simulink model "ccc_core"  (Simulink 7.4)
settings: Solver=ode45  StartTime=0.0  StopTime=10000  RelTol=1e-3
libraries: xbsIndex_r4 x236, cfa_library x64, casper_library_misc x7
(part 3 of 5)

== system ccc_core/ccc_core/real_bram_vacc ==
  new_acc : Inport  OutDataType=sfix(16)  OutScaling=2^0
  din : Inport  Port=2  OutDataType=sfix(16)  OutScaling=2^0
  Adder : xbsIndex_r4/AddSub  mode=Addition  use_carryin=off  use_carryout=off  en=off  latency=add_latency  precision=User Defined  arith_type="Signed  (2's comp)"  n_bits=n_bits  bin_pt=bin_pt  quantization=Truncate  overflow=Wrap  dbl_ovrd=off  use_behavioral_HDL=off  hw_selection=Fabric  pipelined=on  use_rpm=on  block_type=addsub
      settings: xl_area=[0, 0, 0, 0, 0, 0, 0]  block_version=10.1.3
  Constant : xbsIndex_r4/Constant  arith_type=Signed (2's comp)  const=0  n_bits=n_bits  bin_pt=bin_pt  explicit_period=on  period=1  equ=P=C  opselect=C  inp2=PCIN>>17  opr=+  inp1=P  carry=CIN  dbl_ovrd=off  block_type=constant
  Mux : xbsIndex_r4/Mux  inputs=2  en=off  latency=0  precision=Full  arith_type="Signed  (2's comp)"  n_bits=8  bin_pt=2  quantization=Truncate  overflow=Wrap  dbl_ovrd=off  block_type=mux
      settings: xl_area=[0, 0, 0, 0, 0, 0, 0]
  delay_bram : Subsystem  mask(delay_bram){DelayLen=vec_len - add_latency, bram_latency=add_latency}
      mask prompts: DelayLen "Delay By:"; bram_latency "BRAM Latency"
      mask help: A delay block that uses BRAM for its storage.
      mask init:
      | if (DelayLen <= bram_latency)
      | 	error('delay value must be greater than BRAM Latency');
      | end
      | BitWidth = max(ceil(log2(DelayLen)), 2);
      mask Help: eval('xlWeb(''http://casper.berkeley.edu/wiki/Delay_bram'')')
  pulse_ext : Subsystem  mask(pulse_ext){pulse_len=vec_len}
      mask prompts: pulse_len "Length of Pulse"
      mask help:
      | Extends a boolean signal to be high for the specified number of clocks after
      | the last high input.
      mask init:
      | bits = ceil(log2(pulse_len+1));
      mask Help: eval('xlWeb(''http://casper.berkeley.edu/wiki/Pulse_ext'')')
  dout : Outport  OutDataType=sfix(16)  OutScaling=2^0
  valid : Outport  Port=2  OutDataType=sfix(16)  OutScaling=2^0
  wires:
  Adder/1 -> delay_bram/1(In1)
  delay_bram/1(Out1) -> dout/1, Mux/2
  new_acc/1 -> pulse_ext/1(in)
  din/1 -> Adder/1
  pulse_ext/1(out) -> Mux/1, valid/1
  Mux/1 -> Adder/2
  Constant/1 -> Mux/3

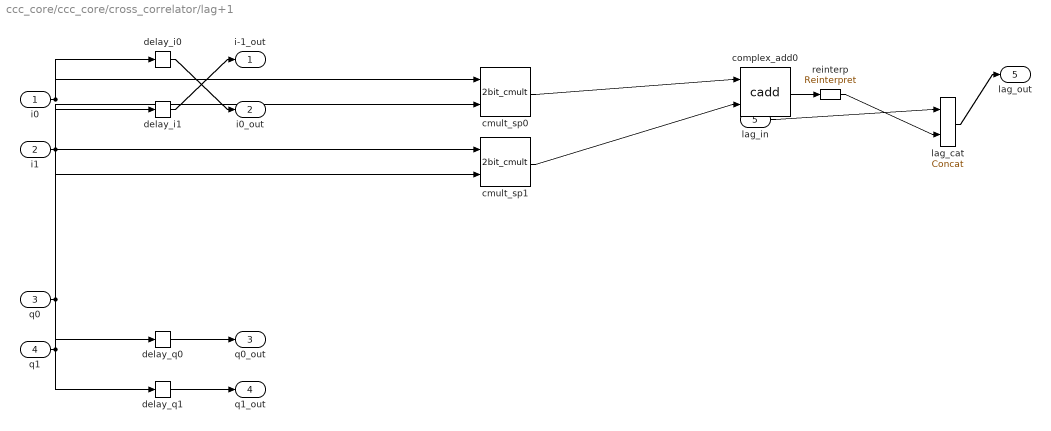
== system ccc_core/ccc_core/cross_correlator/lag+1 ==
  i0 : Inport
  i1 : Inport  Port=2
  q0 : Inport  Port=3
  q1 : Inport  Port=4
  lag_in : Inport  Port=5
  cmult_sp0 : cfa_library/2bit_cmult  SystemSampleTime=-1  add_delay=2
  cmult_sp1 : cfa_library/2bit_cmult  SystemSampleTime=-1  add_delay=2
  complex_add0 : cfa_library/cadd  SystemSampleTime=-1  input_bit_width=6  input_bin_pt=0  add_delay=2
  delay_i0 : xbsIndex_r4/Delay  en=off  latency=2  dbl_ovrd=off  reg_retiming=off  block_type=delay
      settings: block_version=11.4
  delay_i1 : xbsIndex_r4/Delay  en=off  latency=3  dbl_ovrd=off  reg_retiming=off  block_type=delay
      settings: block_version=11.4
  delay_q0 : xbsIndex_r4/Delay  en=off  latency=2  dbl_ovrd=off  reg_retiming=off  block_type=delay
      settings: block_version=11.4
  delay_q1 : xbsIndex_r4/Delay  en=off  latency=2  dbl_ovrd=off  reg_retiming=off  block_type=delay
      settings: block_version=11.4
  lag_cat : xbsIndex_r4/Concat  num_inputs=2  dbl_ovrd=off  block_type=concat
  reinterp : xbsIndex_r4/Reinterpret  force_arith_type=on  arith_type=Unsigned  force_bin_pt=on  bin_pt=0  block_type=reinterpret
      settings: infoedit="Changes signal type without altering the binary representation.   You can changed the signal between signed and unsigned, and relocate the binary point.<br><br>Hardware notes: In hardware this block costs nothing.<br><br>Example:  Suppose the input is 6 bits wide, signed, with 2 fractional bits, and the output is forced to unsigned with 0 fractional bits.  Then an input of -2.0 (1110.00 in binary 2's complement) becomes an output of 56 (111000 in binary)."
  i-1_out : Outport
  i0_out : Outport  Port=2
  q0_out : Outport  Port=3
  q1_out : Outport  Port=4
  lag_out : Outport  Port=5
  wires:
  i0/1 -> cmult_sp0/1, delay_i0/1
  q0/1 -> cmult_sp0/2, delay_q0/1
  i1/1 -> cmult_sp1/1, delay_i1/1
  q1/1 -> cmult_sp1/2, delay_q1/1
  cmult_sp0/1 -> complex_add0/1
  cmult_sp1/1 -> complex_add0/2
  delay_i0/1 -> i0_out/1
  delay_q0/1 -> q0_out/1
  delay_i1/1 -> i-1_out/1
  delay_q1/1 -> q1_out/1
  lag_in/1 -> lag_cat/1
  complex_add0/1 -> reinterp/1
  reinterp/1 -> lag_cat/2
  lag_cat/1 -> lag_out/1

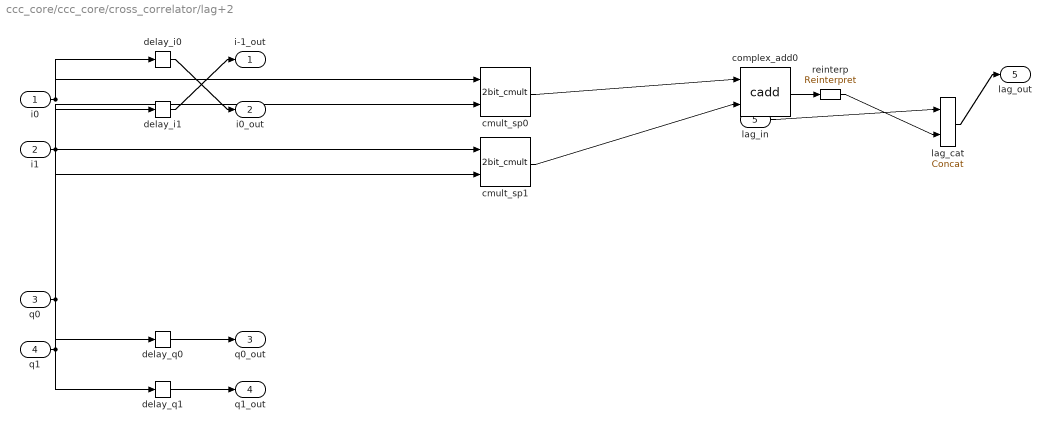
== system ccc_core/ccc_core/cross_correlator/lag+2 ==
  i0 : Inport
  i1 : Inport  Port=2
  q0 : Inport  Port=3
  q1 : Inport  Port=4
  lag_in : Inport  Port=5
  cmult_sp0 : cfa_library/2bit_cmult  SystemSampleTime=-1  add_delay=2
  cmult_sp1 : cfa_library/2bit_cmult  SystemSampleTime=-1  add_delay=2
  complex_add0 : cfa_library/cadd  SystemSampleTime=-1  input_bit_width=6  input_bin_pt=0  add_delay=2
  delay_i0 : xbsIndex_r4/Delay  en=off  latency=2  dbl_ovrd=off  reg_retiming=off  block_type=delay
      settings: block_version=11.4
  delay_i1 : xbsIndex_r4/Delay  en=off  latency=3  dbl_ovrd=off  reg_retiming=off  block_type=delay
      settings: block_version=11.4
  delay_q0 : xbsIndex_r4/Delay  en=off  latency=2  dbl_ovrd=off  reg_retiming=off  block_type=delay
      settings: block_version=11.4
  delay_q1 : xbsIndex_r4/Delay  en=off  latency=2  dbl_ovrd=off  reg_retiming=off  block_type=delay
      settings: block_version=11.4
  lag_cat : xbsIndex_r4/Concat  num_inputs=2  dbl_ovrd=off  block_type=concat
  reinterp : xbsIndex_r4/Reinterpret  force_arith_type=on  arith_type=Unsigned  force_bin_pt=on  bin_pt=0  block_type=reinterpret
      settings: infoedit="Changes signal type without altering the binary representation.   You can changed the signal between signed and unsigned, and relocate the binary point.<br><br>Hardware notes: In hardware this block costs nothing.<br><br>Example:  Suppose the input is 6 bits wide, signed, with 2 fractional bits, and the output is forced to unsigned with 0 fractional bits.  Then an input of -2.0 (1110.00 in binary 2's complement) becomes an output of 56 (111000 in binary)."
  i-1_out : Outport
  i0_out : Outport  Port=2
  q0_out : Outport  Port=3
  q1_out : Outport  Port=4
  lag_out : Outport  Port=5
  wires:
  i0/1 -> cmult_sp0/1, delay_i0/1
  q0/1 -> cmult_sp0/2, delay_q0/1
  i1/1 -> cmult_sp1/1, delay_i1/1
  q1/1 -> cmult_sp1/2, delay_q1/1
  cmult_sp0/1 -> complex_add0/1
  cmult_sp1/1 -> complex_add0/2
  delay_i0/1 -> i0_out/1
  delay_q0/1 -> q0_out/1
  delay_i1/1 -> i-1_out/1
  delay_q1/1 -> q1_out/1
  lag_in/1 -> lag_cat/1
  complex_add0/1 -> reinterp/1
  reinterp/1 -> lag_cat/2
  lag_cat/1 -> lag_out/1

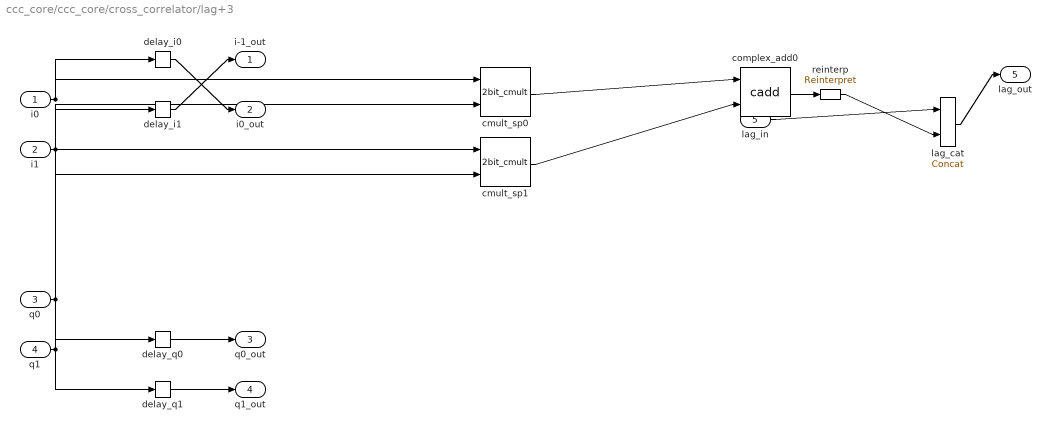
== system ccc_core/ccc_core/cross_correlator/lag+3 ==
  i0 : Inport
  i1 : Inport  Port=2
  q0 : Inport  Port=3
  q1 : Inport  Port=4
  lag_in : Inport  Port=5
  cmult_sp0 : cfa_library/2bit_cmult  SystemSampleTime=-1  add_delay=2
  cmult_sp1 : cfa_library/2bit_cmult  SystemSampleTime=-1  add_delay=2
  complex_add0 : cfa_library/cadd  SystemSampleTime=-1  input_bit_width=6  input_bin_pt=0  add_delay=2
  delay_i0 : xbsIndex_r4/Delay  en=off  latency=2  dbl_ovrd=off  reg_retiming=off  block_type=delay
      settings: block_version=11.4
  delay_i1 : xbsIndex_r4/Delay  en=off  latency=3  dbl_ovrd=off  reg_retiming=off  block_type=delay
      settings: block_version=11.4
  delay_q0 : xbsIndex_r4/Delay  en=off  latency=2  dbl_ovrd=off  reg_retiming=off  block_type=delay
      settings: block_version=11.4
  delay_q1 : xbsIndex_r4/Delay  en=off  latency=2  dbl_ovrd=off  reg_retiming=off  block_type=delay
      settings: block_version=11.4
  lag_cat : xbsIndex_r4/Concat  num_inputs=2  dbl_ovrd=off  block_type=concat
  reinterp : xbsIndex_r4/Reinterpret  force_arith_type=on  arith_type=Unsigned  force_bin_pt=on  bin_pt=0  block_type=reinterpret
      settings: infoedit="Changes signal type without altering the binary representation.   You can changed the signal between signed and unsigned, and relocate the binary point.<br><br>Hardware notes: In hardware this block costs nothing.<br><br>Example:  Suppose the input is 6 bits wide, signed, with 2 fractional bits, and the output is forced to unsigned with 0 fractional bits.  Then an input of -2.0 (1110.00 in binary 2's complement) becomes an output of 56 (111000 in binary)."
  i-1_out : Outport
  i0_out : Outport  Port=2
  q0_out : Outport  Port=3
  q1_out : Outport  Port=4
  lag_out : Outport  Port=5
  wires:
  i0/1 -> cmult_sp0/1, delay_i0/1
  q0/1 -> cmult_sp0/2, delay_q0/1
  i1/1 -> cmult_sp1/1, delay_i1/1
  q1/1 -> cmult_sp1/2, delay_q1/1
  cmult_sp0/1 -> complex_add0/1
  cmult_sp1/1 -> complex_add0/2
  delay_i0/1 -> i0_out/1
  delay_q0/1 -> q0_out/1
  delay_i1/1 -> i-1_out/1
  delay_q1/1 -> q1_out/1
  lag_in/1 -> lag_cat/1
  complex_add0/1 -> reinterp/1
  reinterp/1 -> lag_cat/2
  lag_cat/1 -> lag_out/1

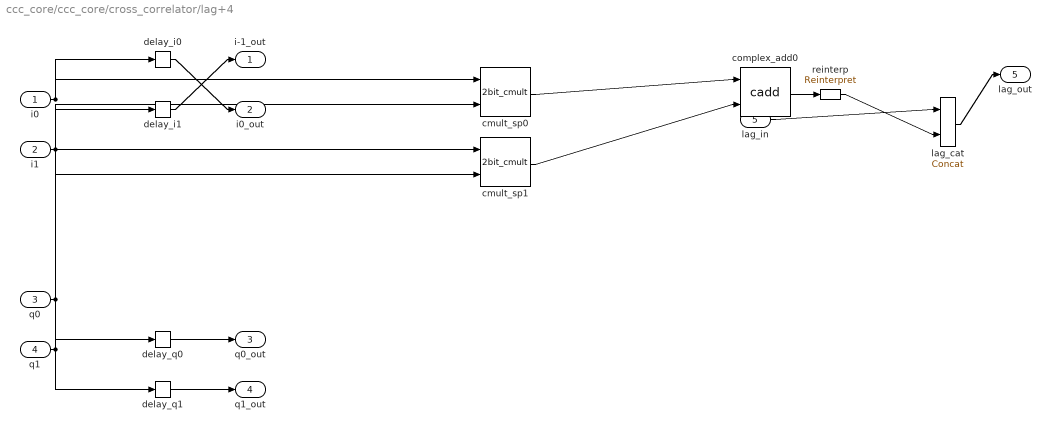
== system ccc_core/ccc_core/cross_correlator/lag+4 ==
  i0 : Inport
  i1 : Inport  Port=2
  q0 : Inport  Port=3
  q1 : Inport  Port=4
  lag_in : Inport  Port=5
  cmult_sp0 : cfa_library/2bit_cmult  SystemSampleTime=-1  add_delay=2
  cmult_sp1 : cfa_library/2bit_cmult  SystemSampleTime=-1  add_delay=2
  complex_add0 : cfa_library/cadd  SystemSampleTime=-1  input_bit_width=6  input_bin_pt=0  add_delay=2
  delay_i0 : xbsIndex_r4/Delay  en=off  latency=2  dbl_ovrd=off  reg_retiming=off  block_type=delay
      settings: block_version=11.4
  delay_i1 : xbsIndex_r4/Delay  en=off  latency=3  dbl_ovrd=off  reg_retiming=off  block_type=delay
      settings: block_version=11.4
  delay_q0 : xbsIndex_r4/Delay  en=off  latency=2  dbl_ovrd=off  reg_retiming=off  block_type=delay
      settings: block_version=11.4
  delay_q1 : xbsIndex_r4/Delay  en=off  latency=2  dbl_ovrd=off  reg_retiming=off  block_type=delay
      settings: block_version=11.4
  lag_cat : xbsIndex_r4/Concat  num_inputs=2  dbl_ovrd=off  block_type=concat
  reinterp : xbsIndex_r4/Reinterpret  force_arith_type=on  arith_type=Unsigned  force_bin_pt=on  bin_pt=0  block_type=reinterpret
      settings: infoedit="Changes signal type without altering the binary representation.   You can changed the signal between signed and unsigned, and relocate the binary point.<br><br>Hardware notes: In hardware this block costs nothing.<br><br>Example:  Suppose the input is 6 bits wide, signed, with 2 fractional bits, and the output is forced to unsigned with 0 fractional bits.  Then an input of -2.0 (1110.00 in binary 2's complement) becomes an output of 56 (111000 in binary)."
  i-1_out : Outport
  i0_out : Outport  Port=2
  q0_out : Outport  Port=3
  q1_out : Outport  Port=4
  lag_out : Outport  Port=5
  wires:
  i0/1 -> cmult_sp0/1, delay_i0/1
  q0/1 -> cmult_sp0/2, delay_q0/1
  i1/1 -> cmult_sp1/1, delay_i1/1
  q1/1 -> cmult_sp1/2, delay_q1/1
  cmult_sp0/1 -> complex_add0/1
  cmult_sp1/1 -> complex_add0/2
  delay_i0/1 -> i0_out/1
  delay_q0/1 -> q0_out/1
  delay_i1/1 -> i-1_out/1
  delay_q1/1 -> q1_out/1
  lag_in/1 -> lag_cat/1
  complex_add0/1 -> reinterp/1
  reinterp/1 -> lag_cat/2
  lag_cat/1 -> lag_out/1

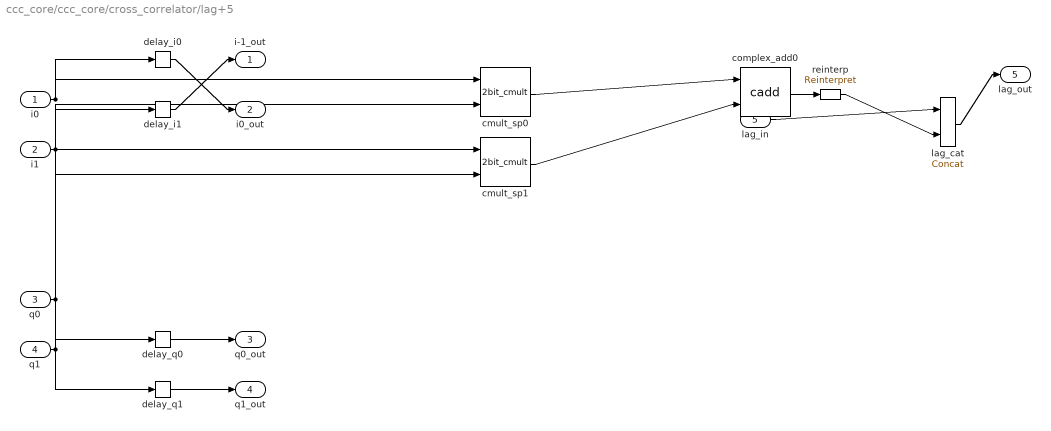
== system ccc_core/ccc_core/cross_correlator/lag+5 ==
  i0 : Inport
  i1 : Inport  Port=2
  q0 : Inport  Port=3
  q1 : Inport  Port=4
  lag_in : Inport  Port=5
  cmult_sp0 : cfa_library/2bit_cmult  SystemSampleTime=-1  add_delay=2
  cmult_sp1 : cfa_library/2bit_cmult  SystemSampleTime=-1  add_delay=2
  complex_add0 : cfa_library/cadd  SystemSampleTime=-1  input_bit_width=6  input_bin_pt=0  add_delay=2
  delay_i0 : xbsIndex_r4/Delay  en=off  latency=2  dbl_ovrd=off  reg_retiming=off  block_type=delay
      settings: block_version=11.4
  delay_i1 : xbsIndex_r4/Delay  en=off  latency=3  dbl_ovrd=off  reg_retiming=off  block_type=delay
      settings: block_version=11.4
  delay_q0 : xbsIndex_r4/Delay  en=off  latency=2  dbl_ovrd=off  reg_retiming=off  block_type=delay
      settings: block_version=11.4
  delay_q1 : xbsIndex_r4/Delay  en=off  latency=2  dbl_ovrd=off  reg_retiming=off  block_type=delay
      settings: block_version=11.4
  lag_cat : xbsIndex_r4/Concat  num_inputs=2  dbl_ovrd=off  block_type=concat
  reinterp : xbsIndex_r4/Reinterpret  force_arith_type=on  arith_type=Unsigned  force_bin_pt=on  bin_pt=0  block_type=reinterpret
      settings: infoedit="Changes signal type without altering the binary representation.   You can changed the signal between signed and unsigned, and relocate the binary point.<br><br>Hardware notes: In hardware this block costs nothing.<br><br>Example:  Suppose the input is 6 bits wide, signed, with 2 fractional bits, and the output is forced to unsigned with 0 fractional bits.  Then an input of -2.0 (1110.00 in binary 2's complement) becomes an output of 56 (111000 in binary)."
  i-1_out : Outport
  i0_out : Outport  Port=2
  q0_out : Outport  Port=3
  q1_out : Outport  Port=4
  lag_out : Outport  Port=5
  wires:
  i0/1 -> cmult_sp0/1, delay_i0/1
  q0/1 -> cmult_sp0/2, delay_q0/1
  i1/1 -> cmult_sp1/1, delay_i1/1
  q1/1 -> cmult_sp1/2, delay_q1/1
  cmult_sp0/1 -> complex_add0/1
  cmult_sp1/1 -> complex_add0/2
  delay_i0/1 -> i0_out/1
  delay_q0/1 -> q0_out/1
  delay_i1/1 -> i-1_out/1
  delay_q1/1 -> q1_out/1
  lag_in/1 -> lag_cat/1
  complex_add0/1 -> reinterp/1
  reinterp/1 -> lag_cat/2
  lag_cat/1 -> lag_out/1

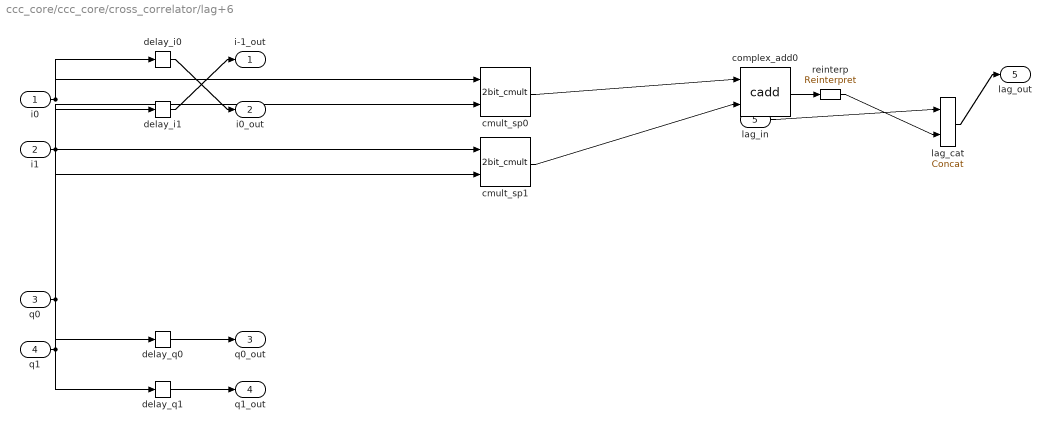
== system ccc_core/ccc_core/cross_correlator/lag+6 ==
  i0 : Inport
  i1 : Inport  Port=2
  q0 : Inport  Port=3
  q1 : Inport  Port=4
  lag_in : Inport  Port=5
  cmult_sp0 : cfa_library/2bit_cmult  SystemSampleTime=-1  add_delay=2
  cmult_sp1 : cfa_library/2bit_cmult  SystemSampleTime=-1  add_delay=2
  complex_add0 : cfa_library/cadd  SystemSampleTime=-1  input_bit_width=6  input_bin_pt=0  add_delay=2
  delay_i0 : xbsIndex_r4/Delay  en=off  latency=2  dbl_ovrd=off  reg_retiming=off  block_type=delay
      settings: block_version=11.4
  delay_i1 : xbsIndex_r4/Delay  en=off  latency=3  dbl_ovrd=off  reg_retiming=off  block_type=delay
      settings: block_version=11.4
  delay_q0 : xbsIndex_r4/Delay  en=off  latency=2  dbl_ovrd=off  reg_retiming=off  block_type=delay
      settings: block_version=11.4
  delay_q1 : xbsIndex_r4/Delay  en=off  latency=2  dbl_ovrd=off  reg_retiming=off  block_type=delay
      settings: block_version=11.4
  lag_cat : xbsIndex_r4/Concat  num_inputs=2  dbl_ovrd=off  block_type=concat
  reinterp : xbsIndex_r4/Reinterpret  force_arith_type=on  arith_type=Unsigned  force_bin_pt=on  bin_pt=0  block_type=reinterpret
      settings: infoedit="Changes signal type without altering the binary representation.   You can changed the signal between signed and unsigned, and relocate the binary point.<br><br>Hardware notes: In hardware this block costs nothing.<br><br>Example:  Suppose the input is 6 bits wide, signed, with 2 fractional bits, and the output is forced to unsigned with 0 fractional bits.  Then an input of -2.0 (1110.00 in binary 2's complement) becomes an output of 56 (111000 in binary)."
  i-1_out : Outport
  i0_out : Outport  Port=2
  q0_out : Outport  Port=3
  q1_out : Outport  Port=4
  lag_out : Outport  Port=5
  wires:
  i0/1 -> cmult_sp0/1, delay_i0/1
  q0/1 -> cmult_sp0/2, delay_q0/1
  i1/1 -> cmult_sp1/1, delay_i1/1
  q1/1 -> cmult_sp1/2, delay_q1/1
  cmult_sp0/1 -> complex_add0/1
  cmult_sp1/1 -> complex_add0/2
  delay_i0/1 -> i0_out/1
  delay_q0/1 -> q0_out/1
  delay_i1/1 -> i-1_out/1
  delay_q1/1 -> q1_out/1
  lag_in/1 -> lag_cat/1
  complex_add0/1 -> reinterp/1
  reinterp/1 -> lag_cat/2
  lag_cat/1 -> lag_out/1

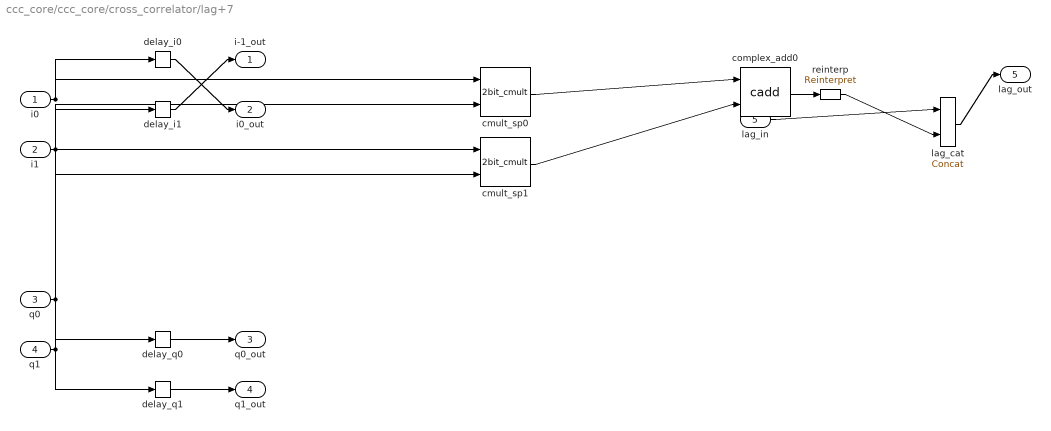
== system ccc_core/ccc_core/cross_correlator/lag+7 ==
  i0 : Inport
  i1 : Inport  Port=2
  q0 : Inport  Port=3
  q1 : Inport  Port=4
  lag_in : Inport  Port=5
  cmult_sp0 : cfa_library/2bit_cmult  SystemSampleTime=-1  add_delay=2
  cmult_sp1 : cfa_library/2bit_cmult  SystemSampleTime=-1  add_delay=2
  complex_add0 : cfa_library/cadd  SystemSampleTime=-1  input_bit_width=6  input_bin_pt=0  add_delay=2
  delay_i0 : xbsIndex_r4/Delay  en=off  latency=2  dbl_ovrd=off  reg_retiming=off  block_type=delay
      settings: block_version=11.4
  delay_i1 : xbsIndex_r4/Delay  en=off  latency=3  dbl_ovrd=off  reg_retiming=off  block_type=delay
      settings: block_version=11.4
  delay_q0 : xbsIndex_r4/Delay  en=off  latency=2  dbl_ovrd=off  reg_retiming=off  block_type=delay
      settings: block_version=11.4
  delay_q1 : xbsIndex_r4/Delay  en=off  latency=2  dbl_ovrd=off  reg_retiming=off  block_type=delay
      settings: block_version=11.4
  lag_cat : xbsIndex_r4/Concat  num_inputs=2  dbl_ovrd=off  block_type=concat
  reinterp : xbsIndex_r4/Reinterpret  force_arith_type=on  arith_type=Unsigned  force_bin_pt=on  bin_pt=0  block_type=reinterpret
      settings: infoedit="Changes signal type without altering the binary representation.   You can changed the signal between signed and unsigned, and relocate the binary point.<br><br>Hardware notes: In hardware this block costs nothing.<br><br>Example:  Suppose the input is 6 bits wide, signed, with 2 fractional bits, and the output is forced to unsigned with 0 fractional bits.  Then an input of -2.0 (1110.00 in binary 2's complement) becomes an output of 56 (111000 in binary)."
  i-1_out : Outport
  i0_out : Outport  Port=2
  q0_out : Outport  Port=3
  q1_out : Outport  Port=4
  lag_out : Outport  Port=5
  wires:
  i0/1 -> cmult_sp0/1, delay_i0/1
  q0/1 -> cmult_sp0/2, delay_q0/1
  i1/1 -> cmult_sp1/1, delay_i1/1
  q1/1 -> cmult_sp1/2, delay_q1/1
  cmult_sp0/1 -> complex_add0/1
  cmult_sp1/1 -> complex_add0/2
  delay_i0/1 -> i0_out/1
  delay_q0/1 -> q0_out/1
  delay_i1/1 -> i-1_out/1
  delay_q1/1 -> q1_out/1
  lag_in/1 -> lag_cat/1
  complex_add0/1 -> reinterp/1
  reinterp/1 -> lag_cat/2
  lag_cat/1 -> lag_out/1

== system ccc_core/ccc_core/cross_correlator/lag-1 ==
  i0 : Inport
  i1 : Inport  Port=2
  q0 : Inport  Port=3
  q1 : Inport  Port=4
  lag_in : Inport  Port=5
  cmult_sp0 : cfa_library/2bit_cmult  SystemSampleTime=-1  add_delay=2
  cmult_sp1 : cfa_library/2bit_cmult  SystemSampleTime=-1  add_delay=2
  complex_add0 : cfa_library/cadd  SystemSampleTime=-1  input_bit_width=6  input_bin_pt=0  add_delay=2
  delay_i0 : xbsIndex_r4/Delay  en=off  latency=2  dbl_ovrd=off  reg_retiming=off  block_type=delay
      settings: block_version=11.4
  delay_i1 : xbsIndex_r4/Delay  en=off  latency=3  dbl_ovrd=off  reg_retiming=off  block_type=delay
      settings: block_version=11.4
  delay_q0 : xbsIndex_r4/Delay  en=off  latency=2  dbl_ovrd=off  reg_retiming=off  block_type=delay
      settings: block_version=11.4
  delay_q1 : xbsIndex_r4/Delay  en=off  latency=2  dbl_ovrd=off  reg_retiming=off  block_type=delay
      settings: block_version=11.4
  lag_cat : xbsIndex_r4/Concat  num_inputs=2  dbl_ovrd=off  block_type=concat
  reinterp : xbsIndex_r4/Reinterpret  force_arith_type=on  arith_type=Unsigned  force_bin_pt=on  bin_pt=0  block_type=reinterpret
      settings: infoedit="Changes signal type without altering the binary representation.   You can changed the signal between signed and unsigned, and relocate the binary point.<br><br>Hardware notes: In hardware this block costs nothing.<br><br>Example:  Suppose the input is 6 bits wide, signed, with 2 fractional bits, and the output is forced to unsigned with 0 fractional bits.  Then an input of -2.0 (1110.00 in binary 2's complement) becomes an output of 56 (111000 in binary)."
  i-1_out : Outport
  i0_out : Outport  Port=2
  q0_out : Outport  Port=3
  q1_out : Outport  Port=4
  lag_out : Outport  Port=5
  wires:
  i0/1 -> cmult_sp0/1, delay_i0/1
  q0/1 -> cmult_sp0/2, delay_q0/1
  i1/1 -> cmult_sp1/1, delay_i1/1
  q1/1 -> cmult_sp1/2, delay_q1/1
  cmult_sp0/1 -> complex_add0/1
  cmult_sp1/1 -> complex_add0/2
  delay_i0/1 -> i0_out/1
  delay_q0/1 -> q0_out/1
  delay_i1/1 -> i-1_out/1
  delay_q1/1 -> q1_out/1
  lag_in/1 -> lag_cat/1
  complex_add0/1 -> reinterp/1
  reinterp/1 -> lag_cat/2
  lag_cat/1 -> lag_out/1

== system ccc_core/ccc_core/cross_correlator/lag-2 ==
  i0 : Inport
  i1 : Inport  Port=2
  q0 : Inport  Port=3
  q1 : Inport  Port=4
  lag_in : Inport  Port=5
  cmult_sp0 : cfa_library/2bit_cmult  SystemSampleTime=-1  add_delay=2
  cmult_sp1 : cfa_library/2bit_cmult  SystemSampleTime=-1  add_delay=2
  complex_add0 : cfa_library/cadd  SystemSampleTime=-1  input_bit_width=6  input_bin_pt=0  add_delay=2
  delay_i0 : xbsIndex_r4/Delay  en=off  latency=2  dbl_ovrd=off  reg_retiming=off  block_type=delay
      settings: block_version=11.4
  delay_i1 : xbsIndex_r4/Delay  en=off  latency=3  dbl_ovrd=off  reg_retiming=off  block_type=delay
      settings: block_version=11.4
  delay_q0 : xbsIndex_r4/Delay  en=off  latency=2  dbl_ovrd=off  reg_retiming=off  block_type=delay
      settings: block_version=11.4
  delay_q1 : xbsIndex_r4/Delay  en=off  latency=2  dbl_ovrd=off  reg_retiming=off  block_type=delay
      settings: block_version=11.4
  lag_cat : xbsIndex_r4/Concat  num_inputs=2  dbl_ovrd=off  block_type=concat
  reinterp : xbsIndex_r4/Reinterpret  force_arith_type=on  arith_type=Unsigned  force_bin_pt=on  bin_pt=0  block_type=reinterpret
      settings: infoedit="Changes signal type without altering the binary representation.   You can changed the signal between signed and unsigned, and relocate the binary point.<br><br>Hardware notes: In hardware this block costs nothing.<br><br>Example:  Suppose the input is 6 bits wide, signed, with 2 fractional bits, and the output is forced to unsigned with 0 fractional bits.  Then an input of -2.0 (1110.00 in binary 2's complement) becomes an output of 56 (111000 in binary)."
  i-1_out : Outport
  i0_out : Outport  Port=2
  q0_out : Outport  Port=3
  q1_out : Outport  Port=4
  lag_out : Outport  Port=5
  wires:
  i0/1 -> cmult_sp0/1, delay_i0/1
  q0/1 -> cmult_sp0/2, delay_q0/1
  i1/1 -> cmult_sp1/1, delay_i1/1
  q1/1 -> cmult_sp1/2, delay_q1/1
  cmult_sp0/1 -> complex_add0/1
  cmult_sp1/1 -> complex_add0/2
  delay_i0/1 -> i0_out/1
  delay_q0/1 -> q0_out/1
  delay_i1/1 -> i-1_out/1
  delay_q1/1 -> q1_out/1
  lag_in/1 -> lag_cat/1
  complex_add0/1 -> reinterp/1
  reinterp/1 -> lag_cat/2
  lag_cat/1 -> lag_out/1

== system ccc_core/ccc_core/cross_correlator/lag-3 ==
  i0 : Inport
  i1 : Inport  Port=2
  q0 : Inport  Port=3
  q1 : Inport  Port=4
  lag_in : Inport  Port=5
  cmult_sp0 : cfa_library/2bit_cmult  SystemSampleTime=-1  add_delay=2
  cmult_sp1 : cfa_library/2bit_cmult  SystemSampleTime=-1  add_delay=2
  complex_add0 : cfa_library/cadd  SystemSampleTime=-1  input_bit_width=6  input_bin_pt=0  add_delay=2
  delay_i0 : xbsIndex_r4/Delay  en=off  latency=2  dbl_ovrd=off  reg_retiming=off  block_type=delay
      settings: block_version=11.4
  delay_i1 : xbsIndex_r4/Delay  en=off  latency=3  dbl_ovrd=off  reg_retiming=off  block_type=delay
      settings: block_version=11.4
  delay_q0 : xbsIndex_r4/Delay  en=off  latency=2  dbl_ovrd=off  reg_retiming=off  block_type=delay
      settings: block_version=11.4
  delay_q1 : xbsIndex_r4/Delay  en=off  latency=2  dbl_ovrd=off  reg_retiming=off  block_type=delay
      settings: block_version=11.4
  lag_cat : xbsIndex_r4/Concat  num_inputs=2  dbl_ovrd=off  block_type=concat
  reinterp : xbsIndex_r4/Reinterpret  force_arith_type=on  arith_type=Unsigned  force_bin_pt=on  bin_pt=0  block_type=reinterpret
      settings: infoedit="Changes signal type without altering the binary representation.   You can changed the signal between signed and unsigned, and relocate the binary point.<br><br>Hardware notes: In hardware this block costs nothing.<br><br>Example:  Suppose the input is 6 bits wide, signed, with 2 fractional bits, and the output is forced to unsigned with 0 fractional bits.  Then an input of -2.0 (1110.00 in binary 2's complement) becomes an output of 56 (111000 in binary)."
  i-1_out : Outport
  i0_out : Outport  Port=2
  q0_out : Outport  Port=3
  q1_out : Outport  Port=4
  lag_out : Outport  Port=5
  wires:
  i0/1 -> cmult_sp0/1, delay_i0/1
  q0/1 -> cmult_sp0/2, delay_q0/1
  i1/1 -> cmult_sp1/1, delay_i1/1
  q1/1 -> cmult_sp1/2, delay_q1/1
  cmult_sp0/1 -> complex_add0/1
  cmult_sp1/1 -> complex_add0/2
  delay_i0/1 -> i0_out/1
  delay_q0/1 -> q0_out/1
  delay_i1/1 -> i-1_out/1
  delay_q1/1 -> q1_out/1
  lag_in/1 -> lag_cat/1
  complex_add0/1 -> reinterp/1
  reinterp/1 -> lag_cat/2
  lag_cat/1 -> lag_out/1

== system ccc_core/ccc_core/cross_correlator/lag-4 ==
  i0 : Inport
  i1 : Inport  Port=2
  q0 : Inport  Port=3
  q1 : Inport  Port=4
  lag_in : Inport  Port=5
  cmult_sp0 : cfa_library/2bit_cmult  SystemSampleTime=-1  add_delay=2
  cmult_sp1 : cfa_library/2bit_cmult  SystemSampleTime=-1  add_delay=2
  complex_add0 : cfa_library/cadd  SystemSampleTime=-1  input_bit_width=6  input_bin_pt=0  add_delay=2
  delay_i0 : xbsIndex_r4/Delay  en=off  latency=2  dbl_ovrd=off  reg_retiming=off  block_type=delay
      settings: block_version=11.4
  delay_i1 : xbsIndex_r4/Delay  en=off  latency=3  dbl_ovrd=off  reg_retiming=off  block_type=delay
      settings: block_version=11.4
  delay_q0 : xbsIndex_r4/Delay  en=off  latency=2  dbl_ovrd=off  reg_retiming=off  block_type=delay
      settings: block_version=11.4
  delay_q1 : xbsIndex_r4/Delay  en=off  latency=2  dbl_ovrd=off  reg_retiming=off  block_type=delay
      settings: block_version=11.4
  lag_cat : xbsIndex_r4/Concat  num_inputs=2  dbl_ovrd=off  block_type=concat
  reinterp : xbsIndex_r4/Reinterpret  force_arith_type=on  arith_type=Unsigned  force_bin_pt=on  bin_pt=0  block_type=reinterpret
      settings: infoedit="Changes signal type without altering the binary representation.   You can changed the signal between signed and unsigned, and relocate the binary point.<br><br>Hardware notes: In hardware this block costs nothing.<br><br>Example:  Suppose the input is 6 bits wide, signed, with 2 fractional bits, and the output is forced to unsigned with 0 fractional bits.  Then an input of -2.0 (1110.00 in binary 2's complement) becomes an output of 56 (111000 in binary)."
  i-1_out : Outport
  i0_out : Outport  Port=2
  q0_out : Outport  Port=3
  q1_out : Outport  Port=4
  lag_out : Outport  Port=5
  wires:
  i0/1 -> cmult_sp0/1, delay_i0/1
  q0/1 -> cmult_sp0/2, delay_q0/1
  i1/1 -> cmult_sp1/1, delay_i1/1
  q1/1 -> cmult_sp1/2, delay_q1/1
  cmult_sp0/1 -> complex_add0/1
  cmult_sp1/1 -> complex_add0/2
  delay_i0/1 -> i0_out/1
  delay_q0/1 -> q0_out/1
  delay_i1/1 -> i-1_out/1
  delay_q1/1 -> q1_out/1
  lag_in/1 -> lag_cat/1
  complex_add0/1 -> reinterp/1
  reinterp/1 -> lag_cat/2
  lag_cat/1 -> lag_out/1

== system ccc_core/ccc_core/cross_correlator/lag-5 ==
  i0 : Inport
  i1 : Inport  Port=2
  q0 : Inport  Port=3
  q1 : Inport  Port=4
  lag_in : Inport  Port=5
  cmult_sp0 : cfa_library/2bit_cmult  SystemSampleTime=-1  add_delay=2
  cmult_sp1 : cfa_library/2bit_cmult  SystemSampleTime=-1  add_delay=2
  complex_add0 : cfa_library/cadd  SystemSampleTime=-1  input_bit_width=6  input_bin_pt=0  add_delay=2
  delay_i0 : xbsIndex_r4/Delay  en=off  latency=2  dbl_ovrd=off  reg_retiming=off  block_type=delay
      settings: block_version=11.4
  delay_i1 : xbsIndex_r4/Delay  en=off  latency=3  dbl_ovrd=off  reg_retiming=off  block_type=delay
      settings: block_version=11.4
  delay_q0 : xbsIndex_r4/Delay  en=off  latency=2  dbl_ovrd=off  reg_retiming=off  block_type=delay
      settings: block_version=11.4
  delay_q1 : xbsIndex_r4/Delay  en=off  latency=2  dbl_ovrd=off  reg_retiming=off  block_type=delay
      settings: block_version=11.4
  lag_cat : xbsIndex_r4/Concat  num_inputs=2  dbl_ovrd=off  block_type=concat
  reinterp : xbsIndex_r4/Reinterpret  force_arith_type=on  arith_type=Unsigned  force_bin_pt=on  bin_pt=0  block_type=reinterpret
      settings: infoedit="Changes signal type without altering the binary representation.   You can changed the signal between signed and unsigned, and relocate the binary point.<br><br>Hardware notes: In hardware this block costs nothing.<br><br>Example:  Suppose the input is 6 bits wide, signed, with 2 fractional bits, and the output is forced to unsigned with 0 fractional bits.  Then an input of -2.0 (1110.00 in binary 2's complement) becomes an output of 56 (111000 in binary)."
  i-1_out : Outport
  i0_out : Outport  Port=2
  q0_out : Outport  Port=3
  q1_out : Outport  Port=4
  lag_out : Outport  Port=5
  wires:
  i0/1 -> cmult_sp0/1, delay_i0/1
  q0/1 -> cmult_sp0/2, delay_q0/1
  i1/1 -> cmult_sp1/1, delay_i1/1
  q1/1 -> cmult_sp1/2, delay_q1/1
  cmult_sp0/1 -> complex_add0/1
  cmult_sp1/1 -> complex_add0/2
  delay_i0/1 -> i0_out/1
  delay_q0/1 -> q0_out/1
  delay_i1/1 -> i-1_out/1
  delay_q1/1 -> q1_out/1
  lag_in/1 -> lag_cat/1
  complex_add0/1 -> reinterp/1
  reinterp/1 -> lag_cat/2
  lag_cat/1 -> lag_out/1

== system ccc_core/ccc_core/cross_correlator/lag-6 ==
  i0 : Inport
  i1 : Inport  Port=2
  q0 : Inport  Port=3
  q1 : Inport  Port=4
  lag_in : Inport  Port=5
  cmult_sp0 : cfa_library/2bit_cmult  SystemSampleTime=-1  add_delay=2
  cmult_sp1 : cfa_library/2bit_cmult  SystemSampleTime=-1  add_delay=2
  complex_add0 : cfa_library/cadd  SystemSampleTime=-1  input_bit_width=6  input_bin_pt=0  add_delay=2
  delay_i0 : xbsIndex_r4/Delay  en=off  latency=2  dbl_ovrd=off  reg_retiming=off  block_type=delay
      settings: block_version=11.4
  delay_i1 : xbsIndex_r4/Delay  en=off  latency=3  dbl_ovrd=off  reg_retiming=off  block_type=delay
      settings: block_version=11.4
  delay_q0 : xbsIndex_r4/Delay  en=off  latency=2  dbl_ovrd=off  reg_retiming=off  block_type=delay
      settings: block_version=11.4
  delay_q1 : xbsIndex_r4/Delay  en=off  latency=2  dbl_ovrd=off  reg_retiming=off  block_type=delay
      settings: block_version=11.4
  lag_cat : xbsIndex_r4/Concat  num_inputs=2  dbl_ovrd=off  block_type=concat
  reinterp : xbsIndex_r4/Reinterpret  force_arith_type=on  arith_type=Unsigned  force_bin_pt=on  bin_pt=0  block_type=reinterpret
      settings: infoedit="Changes signal type without altering the binary representation.   You can changed the signal between signed and unsigned, and relocate the binary point.<br><br>Hardware notes: In hardware this block costs nothing.<br><br>Example:  Suppose the input is 6 bits wide, signed, with 2 fractional bits, and the output is forced to unsigned with 0 fractional bits.  Then an input of -2.0 (1110.00 in binary 2's complement) becomes an output of 56 (111000 in binary)."
  i-1_out : Outport
  i0_out : Outport  Port=2
  q0_out : Outport  Port=3
  q1_out : Outport  Port=4
  lag_out : Outport  Port=5
  wires:
  i0/1 -> cmult_sp0/1, delay_i0/1
  q0/1 -> cmult_sp0/2, delay_q0/1
  i1/1 -> cmult_sp1/1, delay_i1/1
  q1/1 -> cmult_sp1/2, delay_q1/1
  cmult_sp0/1 -> complex_add0/1
  cmult_sp1/1 -> complex_add0/2
  delay_i0/1 -> i0_out/1
  delay_q0/1 -> q0_out/1
  delay_i1/1 -> i-1_out/1
  delay_q1/1 -> q1_out/1
  lag_in/1 -> lag_cat/1
  complex_add0/1 -> reinterp/1
  reinterp/1 -> lag_cat/2
  lag_cat/1 -> lag_out/1

== system ccc_core/ccc_core/cross_correlator/lag-7 ==
  i0 : Inport
  i1 : Inport  Port=2
  q0 : Inport  Port=3
  q1 : Inport  Port=4
  lag_in : Inport  Port=5
  cmult_sp0 : cfa_library/2bit_cmult  SystemSampleTime=-1  add_delay=2
  cmult_sp1 : cfa_library/2bit_cmult  SystemSampleTime=-1  add_delay=2
  complex_add0 : cfa_library/cadd  SystemSampleTime=-1  input_bit_width=6  input_bin_pt=0  add_delay=2
  delay_i0 : xbsIndex_r4/Delay  en=off  latency=2  dbl_ovrd=off  reg_retiming=off  block_type=delay
      settings: block_version=11.4
  delay_i1 : xbsIndex_r4/Delay  en=off  latency=3  dbl_ovrd=off  reg_retiming=off  block_type=delay
      settings: block_version=11.4
  delay_q0 : xbsIndex_r4/Delay  en=off  latency=2  dbl_ovrd=off  reg_retiming=off  block_type=delay
      settings: block_version=11.4
  delay_q1 : xbsIndex_r4/Delay  en=off  latency=2  dbl_ovrd=off  reg_retiming=off  block_type=delay
      settings: block_version=11.4
  lag_cat : xbsIndex_r4/Concat  num_inputs=2  dbl_ovrd=off  block_type=concat
  reinterp : xbsIndex_r4/Reinterpret  force_arith_type=on  arith_type=Unsigned  force_bin_pt=on  bin_pt=0  block_type=reinterpret
      settings: infoedit="Changes signal type without altering the binary representation.   You can changed the signal between signed and unsigned, and relocate the binary point.<br><br>Hardware notes: In hardware this block costs nothing.<br><br>Example:  Suppose the input is 6 bits wide, signed, with 2 fractional bits, and the output is forced to unsigned with 0 fractional bits.  Then an input of -2.0 (1110.00 in binary 2's complement) becomes an output of 56 (111000 in binary)."
  i-1_out : Outport
  i0_out : Outport  Port=2
  q0_out : Outport  Port=3
  q1_out : Outport  Port=4
  lag_out : Outport  Port=5
  wires:
  i0/1 -> cmult_sp0/1, delay_i0/1
  q0/1 -> cmult_sp0/2, delay_q0/1
  i1/1 -> cmult_sp1/1, delay_i1/1
  q1/1 -> cmult_sp1/2, delay_q1/1
  cmult_sp0/1 -> complex_add0/1
  cmult_sp1/1 -> complex_add0/2
  delay_i0/1 -> i0_out/1
  delay_q0/1 -> q0_out/1
  delay_i1/1 -> i-1_out/1
  delay_q1/1 -> q1_out/1
  lag_in/1 -> lag_cat/1
  complex_add0/1 -> reinterp/1
  reinterp/1 -> lag_cat/2
  lag_cat/1 -> lag_out/1

== system ccc_core/ccc_core/cross_correlator/lag-8 ==
  i0 : Inport
  i1 : Inport  Port=2
  q0 : Inport  Port=3
  q1 : Inport  Port=4
  lag_in : Inport  Port=5
  cmult_sp0 : cfa_library/2bit_cmult  SystemSampleTime=-1  add_delay=2
  cmult_sp1 : cfa_library/2bit_cmult  SystemSampleTime=-1  add_delay=2
  complex_add0 : cfa_library/cadd  SystemSampleTime=-1  input_bit_width=6  input_bin_pt=0  add_delay=2
  delay_i0 : xbsIndex_r4/Delay  en=off  latency=2  dbl_ovrd=off  reg_retiming=off  block_type=delay
      settings: block_version=11.4
  delay_i1 : xbsIndex_r4/Delay  en=off  latency=3  dbl_ovrd=off  reg_retiming=off  block_type=delay
      settings: block_version=11.4
  delay_q0 : xbsIndex_r4/Delay  en=off  latency=2  dbl_ovrd=off  reg_retiming=off  block_type=delay
      settings: block_version=11.4
  delay_q1 : xbsIndex_r4/Delay  en=off  latency=2  dbl_ovrd=off  reg_retiming=off  block_type=delay
      settings: block_version=11.4
  lag_cat : xbsIndex_r4/Concat  num_inputs=2  dbl_ovrd=off  block_type=concat
  reinterp : xbsIndex_r4/Reinterpret  force_arith_type=on  arith_type=Unsigned  force_bin_pt=on  bin_pt=0  block_type=reinterpret
      settings: infoedit="Changes signal type without altering the binary representation.   You can changed the signal between signed and unsigned, and relocate the binary point.<br><br>Hardware notes: In hardware this block costs nothing.<br><br>Example:  Suppose the input is 6 bits wide, signed, with 2 fractional bits, and the output is forced to unsigned with 0 fractional bits.  Then an input of -2.0 (1110.00 in binary 2's complement) becomes an output of 56 (111000 in binary)."
  i-1_out : Outport
  i0_out : Outport  Port=2
  q0_out : Outport  Port=3
  q1_out : Outport  Port=4
  lag_out : Outport  Port=5
  wires:
  i0/1 -> cmult_sp0/1, delay_i0/1
  q0/1 -> cmult_sp0/2, delay_q0/1
  i1/1 -> cmult_sp1/1, delay_i1/1
  q1/1 -> cmult_sp1/2, delay_q1/1
  cmult_sp0/1 -> complex_add0/1
  cmult_sp1/1 -> complex_add0/2
  delay_i0/1 -> i0_out/1
  delay_q0/1 -> q0_out/1
  delay_i1/1 -> i-1_out/1
  delay_q1/1 -> q1_out/1
  lag_in/1 -> lag_cat/1
  complex_add0/1 -> reinterp/1
  reinterp/1 -> lag_cat/2
  lag_cat/1 -> lag_out/1

== system ccc_core/ccc_core/cross_correlator/lag0 ==
  i0 : Inport
  i1 : Inport  Port=2
  q0 : Inport  Port=3
  q1 : Inport  Port=4
  lag_in : Inport  Port=5
  cmult_sp0 : cfa_library/2bit_cmult  SystemSampleTime=-1  add_delay=2
  cmult_sp1 : cfa_library/2bit_cmult  SystemSampleTime=-1  add_delay=2
  complex_add0 : cfa_library/cadd  SystemSampleTime=-1  input_bit_width=6  input_bin_pt=0  add_delay=2
  delay_i0 : xbsIndex_r4/Delay  en=off  latency=2  dbl_ovrd=off  reg_retiming=off  block_type=delay
      settings: block_version=11.4
  delay_i1 : xbsIndex_r4/Delay  en=off  latency=3  dbl_ovrd=off  reg_retiming=off  block_type=delay
      settings: block_version=11.4
  delay_q0 : xbsIndex_r4/Delay  en=off  latency=2  dbl_ovrd=off  reg_retiming=off  block_type=delay
      settings: block_version=11.4
  delay_q1 : xbsIndex_r4/Delay  en=off  latency=2  dbl_ovrd=off  reg_retiming=off  block_type=delay
      settings: block_version=11.4
  lag_cat : xbsIndex_r4/Concat  num_inputs=2  dbl_ovrd=off  block_type=concat
  reinterp : xbsIndex_r4/Reinterpret  force_arith_type=on  arith_type=Unsigned  force_bin_pt=on  bin_pt=0  block_type=reinterpret
      settings: infoedit="Changes signal type without altering the binary representation.   You can changed the signal between signed and unsigned, and relocate the binary point.<br><br>Hardware notes: In hardware this block costs nothing.<br><br>Example:  Suppose the input is 6 bits wide, signed, with 2 fractional bits, and the output is forced to unsigned with 0 fractional bits.  Then an input of -2.0 (1110.00 in binary 2's complement) becomes an output of 56 (111000 in binary)."
  i-1_out : Outport
  i0_out : Outport  Port=2
  q0_out : Outport  Port=3
  q1_out : Outport  Port=4
  lag_out : Outport  Port=5
  wires:
  i0/1 -> cmult_sp0/1, delay_i0/1
  q0/1 -> cmult_sp0/2, delay_q0/1
  i1/1 -> cmult_sp1/1, delay_i1/1
  q1/1 -> cmult_sp1/2, delay_q1/1
  cmult_sp0/1 -> complex_add0/1
  cmult_sp1/1 -> complex_add0/2
  delay_i0/1 -> i0_out/1
  delay_q0/1 -> q0_out/1
  delay_i1/1 -> i-1_out/1
  delay_q1/1 -> q1_out/1
  lag_in/1 -> lag_cat/1
  complex_add0/1 -> reinterp/1
  reinterp/1 -> lag_cat/2
  lag_cat/1 -> lag_out/1
